simulink model "MATLABxuexi05"  (R2016a)
settings: Solver=VariableStepAuto  StartTime=0.0  StopTime=40e-3  RelTol=1e-3
settings Model: Creator=24535  LastModifiedBy=24535

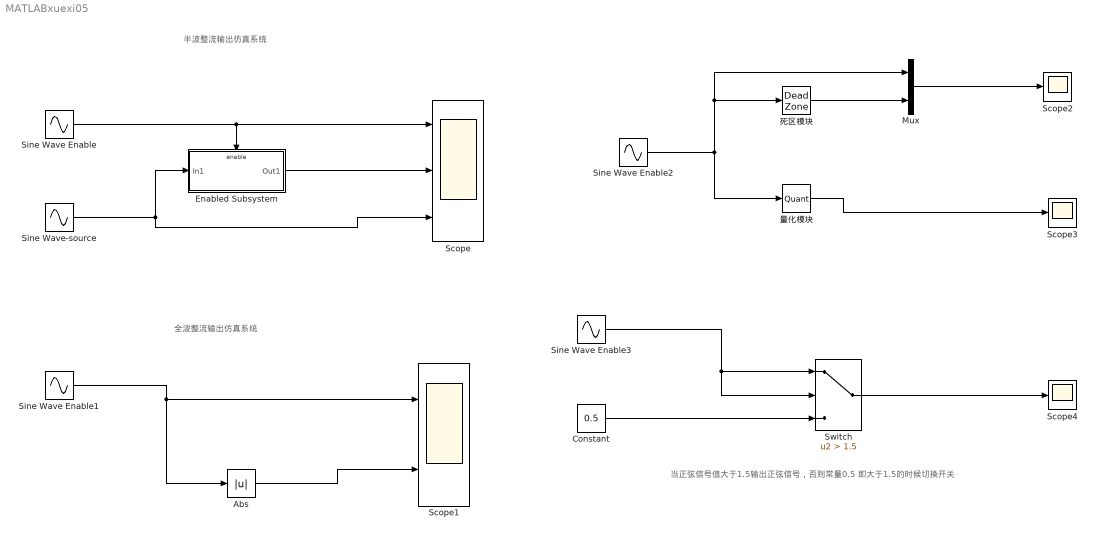
== system MATLABxuexi05 ==
  note: 当正弦信号值大于1.5输出正弦信号，否则常量0.5
      | 即大于1.5的时候切换开关
  note: 半波整流输出仿真系统
  note: 全波整流输出仿真系统
  Abs : Abs
  Constant : Constant  Value=0.5
  Enabled Subsystem : Subsystem  TreatAsAtomicUnit=on
  Mux : Mux  Inputs=2
  Scope : Scope  NumInputPorts=3
  Scope1 : Scope  NumInputPorts=2
  Scope2 : Scope
  Scope3 : Scope
  Scope4 : Scope
  Sine Wave Enable : Sin  Frequency=200*pi  SampleTime=0
  Sine Wave Enable1 : Sin  Frequency=200*pi  SampleTime=0
  Sine Wave Enable2 : Sin  Amplitude=10  Frequency=100*pi  SampleTime=0
  Sine Wave Enable3 : Sin  Amplitude=2  Frequency=100*pi  SampleTime=0
  Sine Wave-source : Sin  Amplitude=220  Frequency=200*pi  SampleTime=0
  Switch : Switch  Criteria=u2 > Threshold  Threshold=1.5
  死区模块 : DeadZone  LowerValue=-5  UpperValue=5  SaturateOnIntegerOverflow=on
  量化模块 : Quantizer  QuantizationInterval=1e-3
  wires:
  Enabled Subsystem/1(Out1) -> Scope/2
  Sine Wave-source/1 -> Enabled Subsystem/1(In1), Scope/3
  Sine Wave Enable/1 -> Enabled Subsystem/Enable, Scope/1
  Sine Wave Enable1/1 -> Scope1/1, Abs/1
  Abs/1 -> Scope1/2
  Sine Wave Enable2/1 -> 死区模块/1, Mux/1, 量化模块/1
  量化模块/1 -> Scope3/1
  Mux/1 -> Scope2/1
  死区模块/1 -> Mux/2
  Constant/1 -> Switch/3
  Sine Wave Enable3/1 -> Switch/1, Switch/2
  Switch/1 -> Scope4/1

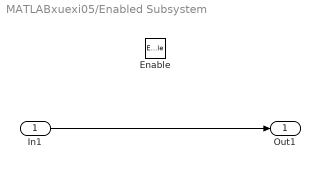
== system MATLABxuexi05/Enabled Subsystem ==
  In1 : Inport
  Enable : EnablePort
  Out1 : Outport
  wires:
  In1/1 -> Out1/1
